simulink model "active_suspension_sim"  (R2013b)
settings: Solver=ode45  StartTime=0.0  StopTime=20.0  MaxStep=0.001  RelTol=1e-3  EnableMultiTasking=on
values from neighbouring files (symbols this model uses):
  A = [[0 1 0 0 0];[-(cw+cs)/mw -ds/mw cs/mw ds/mw -1/mw];[0 0 0 1 0];[cs/mc ds/mc -cs/mc -ds/mc 1/mc];[0 0 0 0 -1/tau]]    [active_suspension_ctrl_design.m]
  B1 = [B H]    [active_suspension_ctrl_design.m]
  C = [[-1 0 1 0 0];[cs/mc ds/mc -cs/mc -ds/mc 1/mc]]    [active_suspension_ctrl_design.m]
  C1 = eye(5)    [active_suspension_ctrl_design.m]
  D1 = zeros(5,2)    [active_suspension_ctrl_design.m]
  K = lqr(A,B,Qx,Qu)    [active_suspension_ctrl_design.m]
settings Model: Creator=JonasMac  LastModifiedBy=JonasMac
settings OptimizationCC: SimCompilerOptimization=off
settings DebuggingCC: FcnCallInpInsideContextMsg=error  FrameProcessingCompatibilityMsg=error  SFExecutionAtInitializationDiag=none
settings HardwareCC: ProdBitPerSizeT=32  ProdBitPerPtrDiffT=32
settings RTWCC: RTWCompilerOptimization=off
settings CodeAppCC: StateflowObjectComments=on
settings GRTTargetCC: TargetLangStandard=C89/C90 (ANSI)  CodeReplacementLibrary=None  CPPClassGenCompliant=on
settings ConfigComp: CovMetricSettings=dw  CovHtmlReporting=on  CovSaveCumulativeToWorkspaceVar=on  CovSaveSingleToWorkspaceVar=on  CovExternalEMLEnable=off

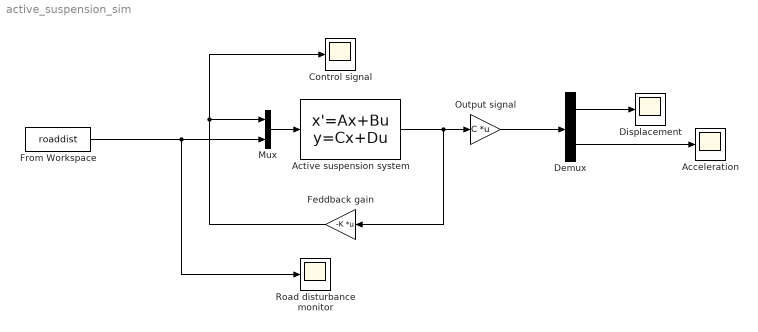
== system active_suspension_sim ==
  Acceleration : Scope
  Active suspension system : StateSpace  A=A  B=B1  C=C1  D=D1
  Control signal : Scope
  Demux : Demux  Outputs=2
  Displacement : Scope
  Feddback gain : Gain  Gain=-K  Multiplication=Matrix(K*u)
  From Workspace : FromWorkspace  VariableName=roaddist  SampleTime=0
  Mux : Mux  Inputs=2
  Output signal : Gain  Gain=C  Multiplication=Matrix(K*u)
  Road disturbance monitor : Scope
  wires:
  Demux/1 -> Displacement/1
  Active suspension system/1 -> Feddback gain/1, Output signal/1
  Feddback gain/1 -> Mux/1, Control signal/1
  Mux/1 -> Active suspension system/1
  Output signal/1 -> Demux/1
  Demux/2 -> Acceleration/1
  From Workspace/1 -> Road disturbance monitor/1, Mux/2
